simulink model "roombaControl"  (R2017b)
settings: Solver=VariableStepAuto  StartTime=0.0  StopTime=inf  RelTol=1e-3
settings Model: Creator=Hoa  LastModifiedBy=Hoa

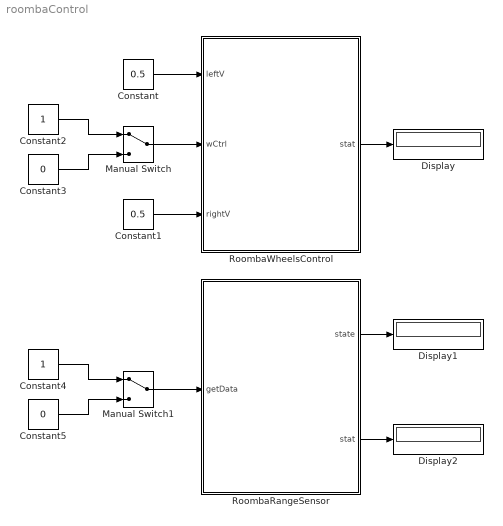
== system roombaControl ==
  Constant : Constant  Value=0.5
  Constant1 : Constant  Value=0.5
  Constant2 : Constant
  Constant3 : Constant  Value=0
  Constant4 : Constant
  Constant5 : Constant  Value=0
  Display : Display
  Display1 : Display
  Display2 : Display
  Manual Switch : ManualSwitch
  Manual Switch1 : ManualSwitch
  RoombaRangeSensor : Subsystem
  RoombaWheelsControl : Subsystem
  wires:
  Constant/1 -> RoombaWheelsControl/1(leftV)
  Constant1/1 -> RoombaWheelsControl/3(rightV)
  Manual Switch/1 -> RoombaWheelsControl/2(wCtrl)
  Constant2/1 -> Manual Switch/1
  Constant3/1 -> Manual Switch/2
  RoombaWheelsControl/1(stat) -> Display/1
  Constant5/1 -> Manual Switch1/2
  Constant4/1 -> Manual Switch1/1
  Manual Switch1/1 -> RoombaRangeSensor/1(getData)
  RoombaRangeSensor/1(state) -> Display1/1
  RoombaRangeSensor/2(stat) -> Display2/1

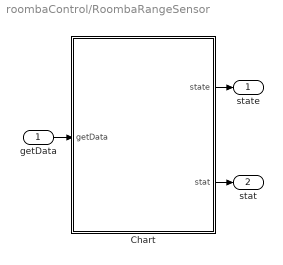
== system roombaControl/RoombaRangeSensor ==
  getData : Inport
  Chart : Stateflow chart  TreatAsAtomicUnit=on
  state : Outport
  stat : Outport  Port=2
  wires:
  getData/1 -> Chart/1(getData)
  Chart/1(state) -> state/1
  Chart/2(stat) -> stat/1

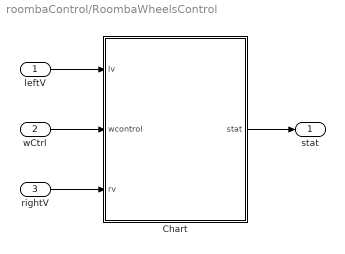
== system roombaControl/RoombaWheelsControl ==
  leftV : Inport
  wCtrl : Inport  Port=2
  rightV : Inport  Port=3
  Chart : Stateflow chart  TreatAsAtomicUnit=on
  stat : Outport
  wires:
  Chart/1(stat) -> stat/1
  wCtrl/1 -> Chart/2(wcontrol)
  leftV/1 -> Chart/1(lv)
  rightV/1 -> Chart/3(rv)

== stateflow chart roombaControl/RoombaRangeSensor/Chart ==
  state NO_OP
    en:
    stat = 0;
  state Reset
    en:
    fwrite(so, 7)
  state START
    en:
    coder.extrinsic('RangeStateRoomba')
    state = RangeStateRoomba('so')
    stat = 1;
  (default) -> NO_OP : {
      | 	coder.extrinsic('RoombaWiFiInit')
      | 	so = RoombaWiFiInit('10.0.0.1','full')
      | }
  Reset -> NO_OP : after(0.1,sec)
  NO_OP -> START : [getData==1]
  START -> Reset : [getData==0]
  data: state output double size=6; stat output; so local; getData input

== stateflow chart roombaControl/RoombaWheelsControl/Chart ==
  state NO_OP
    en:
    stat = 0;
  note: after(1,sec)
  state RESET
    en:
    fwrite(so,7)
  state STOP
    en:
    SetWheelVelRoomba(so,0,0)
  state START
    en:
    coder.extrinsic('SetWheelVelRoomba')
    SetWheelVelRoomba(so,rv,lv)
    stat = 1;
  (default) -> NO_OP : {
      | 	coder.extrinsic('RoombaWiFiInit')
      | 	so = RoombaWiFiInit('10.0.0.1','full')
      | }
  RESET -> NO_OP
  NO_OP -> START : [(wcontrol==1)&&(rv<=0.5||rv>=-0.5)&&(lv<=0.5||lv>=-0.5)]
  STOP -> RESET : [wcontrol==0]
  START -> STOP : after(0.1,sec)
  data: so local; lv input; wcontrol input; rv input; stat output
